simulink model "traffic_generator_sink"  (R2020b)
settings: Solver=ode45  StartTime=0.0  StopTime=10.0  RelTol=1e-3  EnableMultiTasking=on
undefined symbols (not defined in the file or in its folder): SELECT, T
libraries: simulink x1
settings Model: Creator=Nejib  LastModifiedBy=Denis
settings DataIOCC: LimitDataPoints=on  SaveFormat=Array  ReturnWorkspaceOutputs=off
settings OptimizationCC: LifeSpan=inf
settings DebuggingCC: SFUnexpectedBacktrackingDiag=warning  SFNoUnconditionalDefaultTransitionDiag=warning  SFExecutionAtInitializationDiag=none  ArithmeticOperatorsInVariantConditions=warning
settings HardwareCC: ProdBitPerPointer=32  ProdBitPerSizeT=32  ProdBitPerPtrDiffT=32  ProdLargestAtomicFloat=None  ProdIntDivRoundTo=Undefined  ProdEndianess=Unspecified  ProdWordSize=32  ProdHWDeviceType=32-bit Generic
settings ModelReferenceCC: PropagateSignalLabelsOutOfModel=off
settings SFSimCC: SimUseLocalCustomCode=off  CustomCodeUndefinedFunction=UseInterfaceOnly
settings RTWCC: RTWUseLocalCustomCode=off
settings CodeAppCC: StateflowObjectComments=on
settings GRTTargetCC: TargetLangStandard=C89/C90 (ANSI)
settings ConfigComp: CovMetricSettings=dw  CovSaveCumulativeToWorkspaceVar=on  CovSaveSingleToWorkspaceVar=on  CovExternalEMLEnable=off

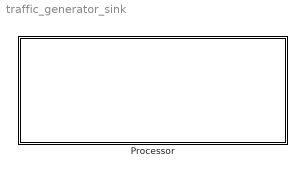
== system traffic_generator_sink ==
  Processor : Subsystem  mask{ME=1, D=5, SEED=100, tt=Periodic, MINU=10, MAXU=200, REGULAR=T, A=100, B=15, Inst='Inst1', Router='Mean1', Loss='Loss1', N='N1'}
      mask prompts: ME "Adress"; D "Startup time"; tt "Traffic Type"; MINU "Min"; MAXU "Max"; REGULAR "T"; A "Lambda 1"; B "Lambda 2"; Inst "Instant delay"; Router "Mean delay"; Loss "Instant number of lost flits"; N "Number of departed flits"
      mask init:
      | set_param([gcb '/Inst'],'VariableName',Inst)
      | set_param([gcb '/Router'],'VariableName',Router)
      | set_param([gcb '/Loss'],'VariableName',Loss)
      | set_param([gcb '/N'],'VariableName',N)
      | V=[2 7 13];
      | %V=1:20;
      | %V=V(V~=ME);
      mask TypeOptions tt: Periodic | Uniform | MMPP
      mask Callback tt:
      | maskStr = get_param(gcb,'tt');
      | msk = Simulink.Mask.get(gcbh);
      | %p = msk.Parameters;
      | %
      | % P = msk.getParameter('MINU');
      | % U = msk.getParameter('MAXU');
      | % M = msk.getParameter('REGULAR');
      | 
      | P = msk.getDialogControl('Periodic');
      | U = msk.getDialogControl('Uniform');
      | M = msk.getDialogControl('MMPP');
      | 
      | % The pop-up menu is the first mask parameter.
      | %   Check the value selected in the pop-up
      | if strcmp(maskStr(1),'P'),
      | 
      |     % Set the visibility of both parameters on when
      |     %   User-defined is selected in the pop-up.
      |     %set_param(gcb,'MaskValues',{'Default','1','1'})
      |     %set_param(gcb,'MaskVisibilities','off'),
      |     SELECT = 1;
      |     P.Visible= 'on';
      |     U.Visible= 'off';
      |     M.Visible= 'off';
      | 
      | elseif strcmp(maskStr(1),'U'),
      |     P.Visible= 'off';
      |     U.Visible= 'on';
      |     M.Visible= 'off';
      | 
      |     SELECT = 2;
      | else
      |     P.Visible= 'off';
      |     U.Visible= 'off';
      |     M.Visible= 'on';
      | 
      |     SELECT = 3;
      | end
      mask DialogControl DescGroupVar Prompt: Processing Element
      mask DialogControl DescTextVar Prompt: Generates traffic from a given adress using one of three possible traffic patterns: Periodic, Uniform and Markov Modulated Poisson Process.
      mask DialogControl Container3 Prompt: Parameters
      mask DialogControl Uniform Prompt: Uniform
      mask DialogControl Periodic Prompt: Periodic
      mask DialogControl MMPP Prompt: MMPP
      mask DialogControl Container7 Prompt: Output Variables

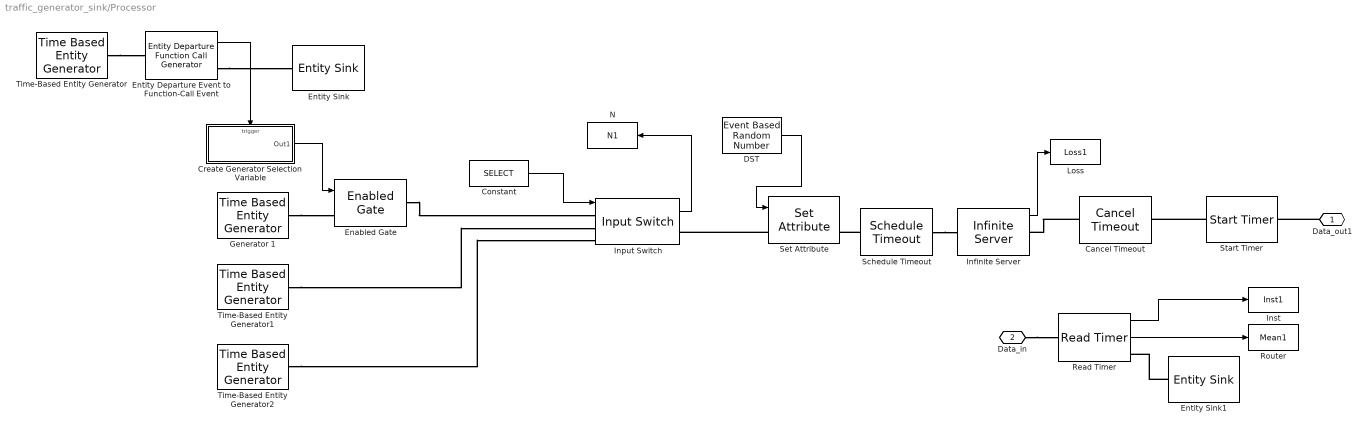
== system traffic_generator_sink/Processor ==
  Cancel Timeout : CancelTimeout
  Constant : Constant  Value=SELECT
  Create Generator Selection Variable : Subsystem  TreatAsAtomicUnit=on
  DST : EventBasedRandomNumber  Distribution=Arbitrary discrete  minUnid=1  maxUnid=16  numValueUnid=5  valueVecDisc=V  probVecDisc=ones(1,3)./3  Seed=SEED+5
  Enabled Gate : EnabledGate
  Entity Departure Event to Function-Call Event : EntityDepartureFunctionCallGenerator
  Entity Sink : EntitySink
  Entity Sink1 : EntitySink
  Generator 1 : TimeBasedEntityGenerator  Distribution=Exponential  Period=.1  InitialSeed=SEED+10  Maximum=.2  Mean=B  ResponseWhenUnblocked=Delayed restart  EntityType=Standard
  Infinite Server : InfiniteServer  ServiceTime=D  EnableTOPort=on  StatNumberTimedout=on
      settings: OutputPortMap=o5
  Input Switch : InputSwitch  SwitchingCriterion=From signal port p  StatNumberDeparted=on
  Inst : ToWorkspace  VariableName=Inst1  SaveFormat=Timeseries  SampleTime=-1
  Loss : ToWorkspace  VariableName=Loss1  SaveFormat=Timeseries  SampleTime=-1
  N : ToWorkspace  VariableName=N1  SaveFormat=Timeseries  SampleTime=-1
  Read Timer : ReadTimer  TimerTag=Departure  StatTimeElapsed=on  StatAverageTimeElapsed=on
      settings: OutputPortMap=o2,o3
  Router : ToWorkspace  VariableName=Mean1  SaveFormat=Timeseries  SampleTime=-1
  Schedule Timeout : ScheduleTimeout  TimeoutInterval=D
  Set Attribute : SetAttribute  AttributeName=DST|SRC  AttributeFrom=Signal port|Dialog  AttributeValue=16|1  AttributeTreatAsVector=0|0  StatNumberDeparted=on  EvaluatedAttributeValue={ [];1}
  Start Timer : StartTimer  TimerTag=Departure
  Time-Based Entity Generator : TimeBasedEntityGenerator  Distribution=Exponential  Period=15  InitialSeed=SEED  Maximum=2  Mean=A  PriorityEntityGeneration=350  EntityType=Standard
  Time-Based Entity Generator1 : TimeBasedEntityGenerator  Period=REGULAR
  Time-Based Entity Generator2 : TimeBasedEntityGenerator  Distribution=Uniform  InitialSeed=SEED  Minimum=MINU  Maximum=MAXU
  Data_out1 : PMIOPort  Side=Right
  Data_in : PMIOPort  Port=2  Side=Left
  wires:
  Create Generator Selection Variable/1(Out1) -> Enabled Gate/1
  Entity Departure Event to Function-Call Event/1 -> Create Generator Selection Variable/Trigger
  Constant/1 -> Input Switch/1
  DST/1 -> Set Attribute/1
  Read Timer/1 -> Inst/1
  Read Timer/2 -> Router/1
  Input Switch/1 -> N/1
  Infinite Server/1 -> Loss/1
  connections:
  Entity Departure Event to Function-Call Event/RConn1 -- Entity Sink/LConn1
  Time-Based Entity Generator/RConn1 -- Entity Departure Event to Function-Call Event/LConn1
  Generator 1/RConn1 -- Enabled Gate/LConn1
  Schedule Timeout/LConn1 -- Set Attribute/RConn1
  Cancel Timeout/LConn1 -- Infinite Server/RConn1
  Set Attribute/LConn1 -- Input Switch/RConn1
  Data_out1/RConn1 -- Start Timer/RConn1
  Start Timer/LConn1 -- Cancel Timeout/RConn1
  Entity Sink1/LConn1 -- Read Timer/RConn1
  Data_in/RConn1 -- Read Timer/LConn1
  Schedule Timeout/RConn1 -- Infinite Server/LConn1
  Time-Based Entity Generator2/RConn1 -- Input Switch/LConn3
  Time-Based Entity Generator1/RConn1 -- Input Switch/LConn2
  Enabled Gate/RConn1 -- Input Switch/LConn1

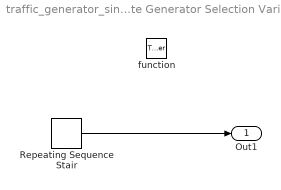
== system traffic_generator_sink/Processor/Create Generator Selection Variable ==
  function : TriggerPort  TriggerType=function-call  VariantControl=(inherit)
  Repeating Sequence Stair : simulink/Sources/Repeating Sequence Stair  OutValues=[0 1].'  tsamp=-1  OutMin=[]  OutMax=[]  OutDataTypeStr=float('double')  OutputDataTypeScalingMode=Specify via dialog  OutDataType=float('double')  ConRadixGroup=Best Precision: Vector-wise  OutScaling=2^-12
  Out1 : Outport
  wires:
  Repeating Sequence Stair/1 -> Out1/1
